simulink model "sim_topic3"  (R2023b)
settings: Solver=FixedStepAuto  StartTime=0.0  StopTime=T_sim  FixedStep=dt_sim  RelTol=1e-3
undefined symbols (not defined in the file): den_Cd_tf, den_Gp_tf, num_Cd_tf, num_Gp_tf, T
settings Model: Creator=user  LastModifiedBy=user

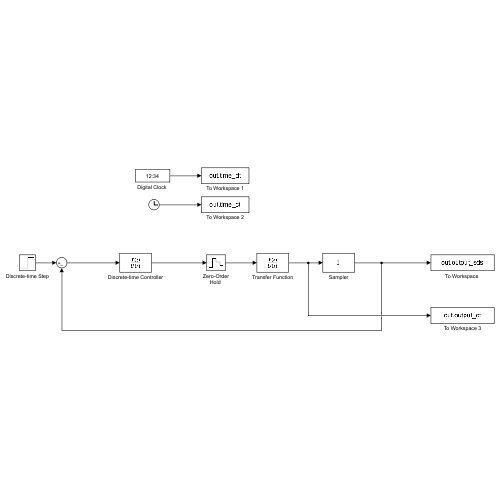
[thumbnail: Simulink's stored preview of the top-level diagram]
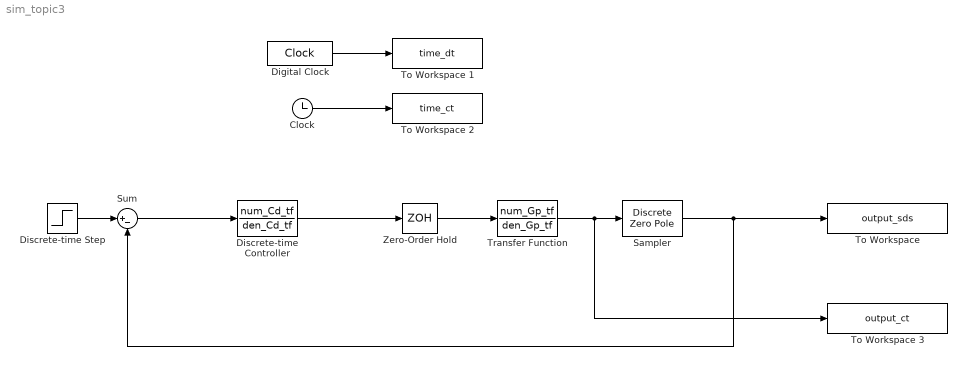
== system sim_topic3 ==
  Clock : Clock
  "Digital Clock " : DigitalClock  SampleTime=T
  Discrete-time Controller : DiscreteTransferFcn  Numerator=num_Cd_tf  Denominator=den_Cd_tf
  Discrete-time Step : Step  Time=0  SampleTime=T
  Sampler : DiscreteZeroPole  Zeros=[]  Poles=[]  Gain=1  SampleTime=T
  Sum : Sum  Inputs=|+-
  "To Workspace " : ToWorkspace  VariableName=output_sds  SampleTime=T
  To Workspace 1 : ToWorkspace  VariableName=time_dt  SampleTime=T
  To Workspace 2 : ToWorkspace  VariableName=time_ct  SampleTime=-1
  To Workspace 3 : ToWorkspace  VariableName=output_ct  SampleTime=-1
  Transfer Function : TransferFcn  Numerator=num_Gp_tf  Denominator=den_Gp_tf
  "Zero-Order Hold " : ZeroOrderHold  SampleTime=-1
  wires:
  Clock/1 -> To Workspace 2/1
  "Zero-Order Hold "/1 -> Transfer Function/1
  "Digital Clock "/1 -> To Workspace 1/1
  Sampler/1 -> "To Workspace "/1, Sum/2
  Transfer Function/1 -> To Workspace 3/1, Sampler/1
  Discrete-time Step/1 -> Sum/1
  Sum/1 -> Discrete-time Controller/1
  Discrete-time Controller/1 -> "Zero-Order Hold "/1
